simulink model "control_pid_lineal"  (R2022b)
settings: Solver=ode45  StartTime=0.0  StopTime=30  MaxStep=0.01  RelTol=1e-3  EnableMultiTasking=on
values from neighbouring files (symbols this model uses):
  K = XX    [codigo_Prac5.m]
  Kp = XX    [codigo_Prac5.m]
  L = XX    [codigo_Prac5.m]
  T = tau    [codigo_Prac5.m]
  Td = XX    [codigo_Prac5.m]
  Ti = XX    [codigo_Prac5.m]
settings Model: Creator=carles  LastModifiedBy=ggarc
settings SolverCC: AlgebraicLoopSolver=TrustRegion
settings DataIOCC: LimitDataPoints=on  SaveFormat=Array  SignalLoggingSaveFormat=ModelDataLogs  ReturnWorkspaceOutputs=off
settings OptimizationCC: ExpressionDepthLimit=2147483647  LifeSpan=inf
settings DebuggingCC: UnderspecifiedInitializationDetection=Classic  MergeDetectMultiDrivingBlocksExec=none  SolverPrmCheckMsg=warning  FcnCallInpInsideContextMsg=warning  UnconnectedInputMsg=warning  UnconnectedOutputMsg=warning  UnconnectedLineMsg=warning  StateNameClashWarn=warning  SFUnexpectedBacktrackingDiag=warning  SFNoUnconditionalDefaultTransitionDiag=warning  SFExecutionAtInitializationDiag=none  SFMachineParentedDataDiag=warning  ArithmeticOperatorsInVariantConditions=warning
settings HardwareCC: ProdBitPerPointer=32  ProdBitPerSizeT=32  ProdBitPerPtrDiffT=32  ProdLargestAtomicFloat=None  ProdIntDivRoundTo=Undefined  ProdEndianess=Unspecified  ProdWordSize=32  ProdHWDeviceType=32-bit Generic
settings ModelReferenceCC: PropagateSignalLabelsOutOfModel=off
settings SFSimCC: SimUseLocalCustomCode=off  CustomCodeUndefinedFunction=UseInterfaceOnly
settings RTWCC: RTWUseLocalCustomCode=off
settings CodeAppCC: StateflowObjectComments=on
settings GRTTargetCC: TargetLangStandard=C89/C90 (ANSI)  CombineOutputUpdateFcns=off  GRTInterface=on
settings ConfigComp: CovMetricSettings=dw  CovSaveCumulativeToWorkspaceVar=on  CovSaveSingleToWorkspaceVar=on  CovExternalEMLEnable=off  CovSFcnEnable=off

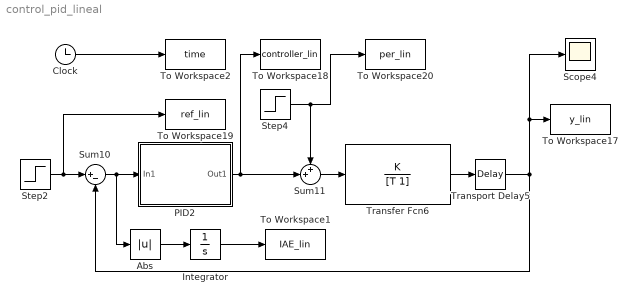
== system control_pid_lineal ==
  Abs : Abs  SaturateOnIntegerOverflow=off
  Clock : Clock
  Integrator : Integrator
  PID2 : Subsystem
  Scope4 : Scope
  Step2 : Step  Time=5  SampleTime=0
  Step4 : Step  Time=30  SampleTime=0
  Sum10 : Sum  Inputs=|+-
  Sum11 : Sum  Inputs=++|
  To Workspace1 : ToWorkspace  VariableName=IAE_lin  SampleTime=-1
  To Workspace17 : ToWorkspace  VariableName=y_lin  SampleTime=-1
  To Workspace18 : ToWorkspace  VariableName=controller_lin  SampleTime=-1
  To Workspace19 : ToWorkspace  VariableName=ref_lin  SampleTime=-1
  To Workspace2 : ToWorkspace  VariableName=time  SaveFormat=Structure With Time  SampleTime=-1
  To Workspace20 : ToWorkspace  VariableName=per_lin  SampleTime=-1
  Transfer Fcn6 : TransferFcn  Numerator=K  Denominator=[T 1]
  Transport Delay5 : TransportDelay  DelayTime=L
  wires:
  Transfer Fcn6/1 -> Transport Delay5/1
  Clock/1 -> To Workspace2/1
  Abs/1 -> Integrator/1
  Integrator/1 -> To Workspace1/1
  Sum10/1 -> Abs/1, PID2/1(In1)
  PID2/1(Out1) -> Sum11/2, To Workspace18/1
  Step2/1 -> To Workspace19/1, Sum10/1
  Step4/1 -> To Workspace20/1, Sum11/1
  Sum11/1 -> Transfer Fcn6/1
  Transport Delay5/1 -> Sum10/2, Scope4/1, To Workspace17/1

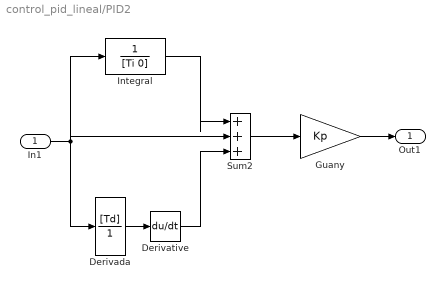
== system control_pid_lineal/PID2 ==
  In1 : Inport
  Derivada : TransferFcn  Numerator=[Td]  Denominator=[1]
  Derivative : Derivative
  Guany : Gain  Gain=Kp
  Integral : TransferFcn  Denominator=[Ti 0]
  Sum2 : Sum  Inputs=|+++
  Out1 : Outport
  wires:
  Guany/1 -> Out1/1
  Sum2/1 -> Guany/1
  Integral/1 -> Sum2/1
  In1/1 -> Sum2/2, Derivada/1, Integral/1
  Derivada/1 -> Derivative/1
  Derivative/1 -> Sum2/3
